simulink model "kalman"  (Simulink 7.1)
settings: Solver=ode45  StartTime=0.0  StopTime=10.0  RelTol=1e-3
settings Model: Creator=claudio  LastModifiedBy=claudio

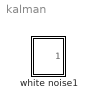
== system kalman ==
  white noise1 : Subsystem  mask(Continuous White Noise.){@1=Rw, @2=0.1, @3=12}
      mask prompts: @1 "Noise Variance:"; @2 "Sample Time:"; @3 "Seed"
      mask help:
      | White noise for continuous (s-domain) systems.
      | Band-limited using zero-order-hold.
      mask init:
      | Cov = @1; Ts = @2; seed = @3;
      mask Help: Implemented using white noise into Zero Order Hold block. For faster simulation set sample time to highest value possible but in accordance with the fastest dynamics of system.
      mask Display: plot(1:20,rand(1,20))

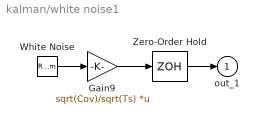
== system kalman/white noise1 ==
  Gain9 : Gain  Gain=sqrt(Cov)/sqrt(Ts)  Multiplication=Matrix(K*u)  ParameterDataType=sfix(16)  ParameterScaling=2^0  OutDataType=sfix(16)  OutScaling=2^0
  White Noise : RandomNumber  Mean=zeros(length(Cov),1)  Variance=ones(length(Cov),1)  Seed=seed
  Zero-Order Hold : ZeroOrderHold  SampleTime=Ts
  out_1 : Outport  OutDataType=sfix(16)  OutScaling=2^0
  wires:
  Zero-Order Hold/1 -> out_1/1
  White Noise/1 -> Gain9/1
  Gain9/1 -> Zero-Order Hold/1
